simulink model "Plant_sim"  (Simulink 7.8)
settings: Solver=FixedStepDiscrete  StartTime=0.0  StopTime=valid_range_time(end)  FixedStep=T_step  RelTol=1e-3
InitFcn:
  | Plant_sim_init
values from neighbouring files (symbols this model uses):
  T_step = 0.01    [boat_constants.m]    (also in common.m)
settings Model: Creator=Bryant  LastModifiedBy=Bryant
settings OptimizationCC: LifeSpan=30

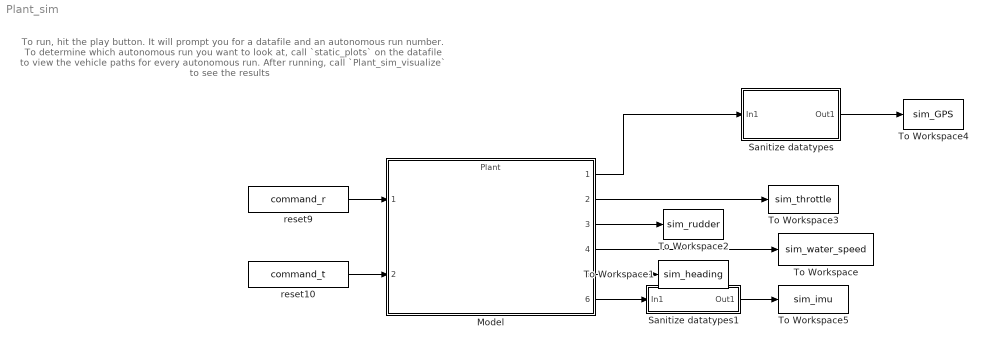
== system Plant_sim ==
  note: To run, hit the play button. It will prompt you for a datafile and an autonomous run number.
      |
      | To determine which autonomous run you want to look at, call `static_plots` on the datafile to
      | view the vehicle paths for every autonomous run.
      |
      | After running, call `Plant_sim_visualize` to see the results
  Model : ModelReference  ModelNameDialog=Plant  SimulationMode=Normal  ModelReferenceVersion=1.40  CopyOfModelName=Plant  DefaultDataLogging=on
  Sanitize datatypes : Subsystem
  Sanitize datatypes1 : Subsystem
  To Workspace : ToWorkspace  VariableName=sim_water_speed  SampleTime=-1  SaveFormat=Structure With Time
  To Workspace1 : ToWorkspace  VariableName=sim_heading  SampleTime=-1  SaveFormat=Structure With Time
  To Workspace2 : ToWorkspace  VariableName=sim_rudder  SampleTime=-1  SaveFormat=Structure With Time
  To Workspace3 : ToWorkspace  VariableName=sim_throttle  SampleTime=-1  SaveFormat=Structure With Time
  To Workspace4 : ToWorkspace  VariableName=sim_GPS  SampleTime=-1  SaveFormat=Structure With Time
  To Workspace5 : ToWorkspace  VariableName=sim_imu  SampleTime=-1  SaveFormat=Structure With Time
  reset10 : FromWorkspace  VariableName=command_t  SampleTime=T_step  Interpolate=off  OutputAfterFinalValue=Holding final value
  reset9 : FromWorkspace  VariableName=command_r  SampleTime=T_step  Interpolate=off  OutputAfterFinalValue=Holding final value
  wires:
  Model/5 -> To Workspace1/1
  Model/4 -> To Workspace/1
  reset9/1 -> Model/1
  reset10/1 -> Model/2
  Model/1 -> Sanitize datatypes/1(In1)
  Model/2 -> To Workspace3/1
  Model/3 -> To Workspace2/1
  Sanitize datatypes/1(Out1) -> To Workspace4/1
  Model/6 -> Sanitize datatypes1/1(In1)
  Sanitize datatypes1/1(Out1) -> To Workspace5/1

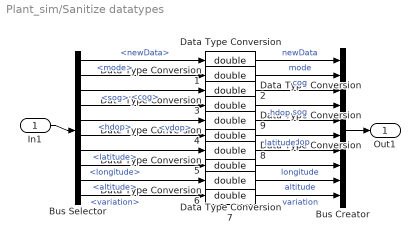
== system Plant_sim/Sanitize datatypes ==
  In1 : Inport
  Bus Creator : BusCreator  Inputs=10
  Bus Selector : BusSelector  OutputSignals=newData,mode,cog,sog,hdop,vdop,latitude,longitude,altitude,variation
  Data Type Conversion{,1..9} (10 alike) : DataTypeConversion  OutDataTypeStr=double  RndMeth=Simplest
  Out1 : Outport
  wires:
  Bus Selector/1 -> Data Type Conversion/1  "<newData>"
  Bus Selector/2 -> Data Type Conversion1/1  "<mode>"
  Data Type Conversion/1 -> Bus Creator/1  "newData"
  Data Type Conversion1/1 -> Bus Creator/2  "mode"
  Bus Selector/3 -> Data Type Conversion2/1  "<cog>"
  Data Type Conversion2/1 -> Bus Creator/3  "cog"
  Bus Selector/4 -> Data Type Conversion3/1  "<sog>"
  Data Type Conversion3/1 -> Bus Creator/4  "sog"
  Bus Selector/5 -> Data Type Conversion9/1  "<hdop>"
  Data Type Conversion9/1 -> Bus Creator/5  "hdop"
  Bus Selector/6 -> Data Type Conversion4/1  "<vdop>"
  Data Type Conversion4/1 -> Bus Creator/6  "vdop"
  Bus Selector/7 -> Data Type Conversion8/1  "<latitude>"
  Data Type Conversion8/1 -> Bus Creator/7  "latitude"
  Bus Selector/8 -> Data Type Conversion5/1  "<longitude>"
  Data Type Conversion5/1 -> Bus Creator/8  "longitude"
  Bus Selector/9 -> Data Type Conversion7/1  "<altitude>"
  Data Type Conversion7/1 -> Bus Creator/9  "altitude"
  Bus Selector/10 -> Data Type Conversion6/1  "<variation>"
  Data Type Conversion6/1 -> Bus Creator/10  "variation"
  In1/1 -> Bus Selector/1
  Bus Creator/1 -> Out1/1

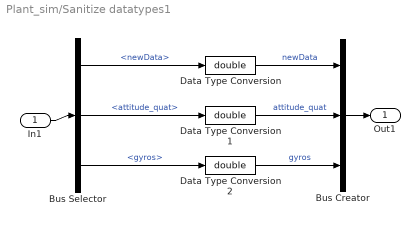
== system Plant_sim/Sanitize datatypes1 ==
  In1 : Inport
  Bus Creator : BusCreator  Inputs=3
  Bus Selector : BusSelector  OutputSignals=newData,attitude_quat,gyros
  Data Type Conversion : DataTypeConversion  OutDataTypeStr=double  RndMeth=Simplest
  Data Type Conversion1 : DataTypeConversion  OutDataTypeStr=double  RndMeth=Simplest
  Data Type Conversion2 : DataTypeConversion  OutDataTypeStr=double  RndMeth=Simplest
  Out1 : Outport
  wires:
  Bus Creator/1 -> Out1/1
  In1/1 -> Bus Selector/1
  Data Type Conversion2/1 -> Bus Creator/3  "gyros"
  Bus Selector/3 -> Data Type Conversion2/1  "<gyros>"
  Data Type Conversion1/1 -> Bus Creator/2  "attitude_quat"
  Data Type Conversion/1 -> Bus Creator/1  "newData"
  Bus Selector/2 -> Data Type Conversion1/1  "<attitude_quat>"
  Bus Selector/1 -> Data Type Conversion/1  "<newData>"
